simulink model "controller_template"  (Simulink 7.8)
settings: Solver=FixedStepDiscrete  SolverMode=SingleTasking  StartTime=0.0  StopTime=inf  FixedStep=Ts  RelTol=1e-3
PreLoadFcn:
  | load_waypoints
  | main;
StopFcn:
  | y_ref_wall = RecordYZ.signals(1).values(:,2);
  | y_wall = RecordYZ.signals(1).values(:,1);
  | 
  | z_ref_wall = RecordYZ.signals(2).values(:,2);
  | z_wall = RecordYZ.signals(2).values(:,1);
  | 
  | close all;
  | figure;
  | plot(y_ref_wall,z_ref_wall,'b','LineWidth',2); hold on;
  | plot(y_wall,z_wall,'r','LineWidth',2); grid on;
  | plot(traj_FG.X_ref_y_real(1,:),-traj_FG.X_ref_z_real(1,:),'o-g');
  | axis equal;
values from neighbouring files (symbols this model uses):
  Add_pitch = [0.764669359834 -6.55628329998 0 0 0.0133529191446 -0.0326334422872 0 0 0 0 0 0 ... (16 elements, 4x4)]    [kostas_malakies.mat]    (also in kostas_malakies2.mat)
  Aff_pitch = [0.764669359834 -6.55628329998 -0.0099932514458 -0.411590904828 0.0133529191446 -0.0326334422872 -8.8646944178e-05 -0.00470014240893 0 0 1 0 ... (16 elements, 4x4)]    [kostas_malakies.mat]    (also in kostas_malakies2.mat)
  Aff_roll = [0.825180563081 -6.10606264808 -0.00763580464276 -0.367448917026 0.0145694646817 0.0253169520582 -6.457583527e-05 -0.00409059128644 0 0 1 0 ... (16 elements, 4x4)]    [kostas_malakies.mat]    (also in kostas_malakies2.mat; main.m = [Aff_roll,zeros(size(Aff_roll,1),1);zeros(1,size(Aff_roll,1); main_last.m = [Aff_roll,zeros(size(Aff_roll,1),1);zeros(1,size(Aff_roll,1))
  Bdd_pitch = [0.235330640166  -0.000506747889746; 6.55628329998  -0.0141179351932; 0  0; 0  0]    [kostas_malakies.mat]    (also in kostas_malakies2.mat)
  Bff_pitch = [0.235330640166  0; 6.55628329998  0; -0.000567656018985  0; -0.0435256495914  0]    [kostas_malakies.mat]    (also in kostas_malakies2.mat)
  Bff_roll = [0.174819436919  0; 6.10606264808  0; -0.000299760068643  0; -0.0270637325616  0]    [kostas_malakies.mat]    (also in kostas_malakies2.mat; main.m = [Bff_roll;zeros(1,size(Bff_roll,2))]; main_last.m = [Bff_roll;zeros(1,size(Bff_roll,2))])
  Fi_Xdir = [-3.0499319419 0 -7.4272134917 -0.3906339295 0 0 -7.4272134917 -1.4749060606 -2.0114272215 -3.0499319419 -7.4272134917 -1.154776828 ... (624 elements, 156x4)]    [kostas_malakies.mat]    (also in kostas_malakies2.mat = [0 0 -2.6412818692 0 0 -3.3089352882 0 -2.6412818692 0 -2.64)
  Fi_XdirFF = [-0.447351940284 0 0 -1.28434394361 -4.04417159595 -1.80654990505 -1.28434394361 1 -4.04417159595 -1.80654990505 1 0 ... (536 elements, 134x4)]    [kostas_malakies.mat]    (also in kostas_malakies2.mat; matlab.mat = [-1.62441280603 -1.28434394361 -1.7723315065 -1.66810627541 )
  Fi_Yaw = [-1.14619813144 0 0]    [kostas_malakies.mat]    (also in kostas_malakies2.mat; matlab.mat = -0.284754025426)
  Fi_Ydir = [-0.466308586531 2.22044604925e-16 2.22044604925e-16 -1.46518332723 -4.54395337171 -2.00318743375 -1.46518332723 1 -4.54395337171 -2.00318743375 1 2.22044604925e-16 ... (536 elements, 134x4)]    [kostas_malakies.mat]    (also in kostas_malakies2.mat = [-0.521298425559 -2.64128186917 -15.6565978667 -8.2066553194; matlab.mat = [1 -1.9173235349 -1.46518332723 1 1 1 1 1 -1.98764774833 -1.)
  Fi_Zdir = [0 -1.80359099426e-16 0 1.4149586889 0 0 2.30859647265e-14 -5.77149118162e-15 0 0 0 0 ... (54 elements, 27x2)]    [kostas_malakies.mat]    (also in kostas_malakies2.mat = [4.30976351396 0 4.73307471514 3.80948040666 0 0 0 0.5468933; matlab.mat = [0 -9.51943523339e-14 0 1.99761158231 0 1.18992940417e-14 0 )
  g = 9.8065    [kostas_malakies.mat]    (also in kostas_malakies2.mat; load_PMModel.m = 9.81; main.m; main_last.m)
  Gi_Xdir = [33.5705355246 -0.267 268.54680224 -0.0188924328 -0.267 -0.267 268.54680224 0.039239647 0.0672163769 0.1708155012 1.343002558 0.0122735546 ... (156 elements, 156x1)]    [kostas_malakies.mat]    (also in kostas_malakies2.mat = [-0.267 -0.267 -1.8623973597 -0.267 -0.267 16.4050483477 -0.)
  Gi_XdirFF = [0 0.27 -0.27 0.478341621792 -6.42962779272 -1.98615606962 -0.478341621792 -0.373552567526 6.42962779272 1.98615606962 0.373552567526 0.27 ... (134 elements, 134x1)]    [kostas_malakies.mat]    (also in kostas_malakies2.mat; matlab.mat = [3.88578058619e-16 0.478341621792 -0.139455879222 -0.1159311)
  Gi_Yaw = [4.4408920985e-16 -3.14159265359 3.14159265359]    [kostas_malakies.mat]    (also in kostas_malakies2.mat = [-4.4408920985e-16 -3.14159265359 3.14159265359]; matlab.mat = 4.4408920985e-16)
  Gi_Ydir = [-2.77555756156e-16 0.27 -0.27 0.516209388722 7.06668201156 2.10835273651 -0.516209388722 -0.383863816771 -7.06668201156 -2.10835273651 0.383863816771 0.27 ... (134 elements, 134x1)]    [kostas_malakies.mat]    (also in kostas_malakies2.mat = [1.11022302463e-16 0.765579126644 531.260413192 11.754237275; matlab.mat = [0.383863816771 -0.133207088705 0.516209388722 0.38386381677)
  Gi_Zdir = [-1 -1 -1 2.22044604925e-16 -1 -1 -1 -1 1 -1 -1 -1 ... (27 elements, 27x1)]    [kostas_malakies.mat]    (also in kostas_malakies2.mat = [0.174387892495 -1 0.368373831608 3.33066907388e-16 -1 -1 -1; matlab.mat = [-2 -2 -2 1.11022302463e-15 -2 -2 -2 2 -2 -2 -2 2 ... (21 el)
  Hn_Xdir = [0.0894044100374 0.0185803675847 -0.0787469077295 -1 0 0.0903062437314 0.0275585020049 -0.0791302456941 -0.0894044100374 -0.0892208721324 -1 0 ... (5248 elements, 1312x4)]    [kostas_malakies.mat]    (also in kostas_malakies2.mat = [0.194772943522 -0.999280166414 0.0919386851603 -0.143548982)
  Hn_XdirFF = [-0.618529611748 0.618529611748 0.827215259158 -0.512155371354 -0.650909395739 -0.827215259158 0.930717154057 0.512155371354 0.650909395739 -0.930717154057 -1 0 ... (4464 elements, 1116x4)]    [kostas_malakies.mat]    (also in kostas_malakies2.mat; matlab.mat = [1 -0.136019433325 -0.405248495598 -0.339279056031 0 -1 0.13)
  Hn_Yaw = [1 -1 -1 1 1 -1]    [kostas_malakies.mat]    (also in kostas_malakies2.mat; matlab.mat = [1 -1])
  Hn_Ydir = [-0.642151612842 0.642151612842 0.873369621238 0.521434628645 0.668917219747 -0.873369621238 0.934789012395 -0.521434628645 -0.668917219747 -0.934789012395 -1 0 ... (4532 elements, 1133x4)]    [kostas_malakies.mat]    (also in kostas_malakies2.mat = [0.972602710123 0.0284063109089 0.559530157965 0.73050130567; matlab.mat = [0.711566553558 0.999813894311 -0.735660470031 0 0 0.5471922)
  Hn_Zdir = [-0.560552458797 -0.996815278536 -0.988320507921 0.666673243042 -1 0 -0.421994354267 -0.987440631917 -0.973284290019 -0.956170964903 -0.936236606521 0.560552458797 ... (224 elements, 112x2)]    [kostas_malakies.mat]    (also in kostas_malakies2.mat = [-0.781813705838 -0.712499731132 0.751798766698 0 -0.7286973; matlab.mat = [1 -1 -0.996815278536 -0.990718937584 -0.276007160242 0.3840)
  kalm_mpc_yaw =     [kostas_malakies.mat]    (also in kostas_malakies2.mat)
  Kn_Xdir = [0.991899150003 0.997410232697 -0.994647298545 0.5094 5 0.992251952723 0.997427328059 -0.992171068824 -0.991899150003 -0.991948411946 0.5094 5 ... (1312 elements, 1312x1)]    [kostas_malakies.mat]    (also in kostas_malakies2.mat = [0.972973501195 0.603589097273 0.988510480824 -0.97816203365)
  Kn_XdirFF = [0.373314565409 0.373314565409 0.472754204418 0.915522246067 0.951154784392 0.472754204418 0.240212330437 0.915522246067 0.951154784392 0.240212330437 0.2094 2 ... (1116 elements, 1116x1)]    [kostas_malakies.mat]    (also in kostas_malakies2.mat; matlab.mat = [0.2094 0.19132523886 0.382063154155 0.900203176458 2 0.2094)
  Kn_Yaw = [2.74088097634 2.74088097634 -2.74088097634 3.14159265359 -2.74088097634 3.14159265359]    [kostas_malakies.mat]    (also in kostas_malakies2.mat; matlab.mat = [0.0873 0.0873])
  Kn_Ydir = [0.371815875743 0.371815875743 0.451349483511 0.90366201682 0.917647772499 0.451349483511 0.24471770913 0.90366201682 0.917647772499 0.24471770913 0.2094 2 ... (1133 elements, 1133x1)]    [kostas_malakies.mat]    (also in kostas_malakies2.mat = [0.351231202126 0.997082913977 0.855763802521 0.792250278627; matlab.mat = [-0.126119149197 0.0536759032179 0.37354703421 2 2 -0.239682)
  Kn_Zdir = [0.727672356179 1.00172267683 1.00656919451 -0.471160923828 1 1 1.18526984431 1.00688561667 1.01272393898 1.01603878926 1.01572683497 -0.727672356179 ... (112 elements, 112x1)]    [kostas_malakies.mat]    (also in kostas_malakies2.mat = [0.21304012328 0.326509029469 -0.262060822346 1 0.301409884 ; matlab.mat = [1 1 1.00663007512 1.02122194908 0.632590992205 -0.384463644)
  MAX_BIAS_YAW_RATE = 0.0872664625997    [kostas_malakies.mat]    (also in kostas_malakies2.mat; main.m; main_last.m)
  Nc_Xdir = [5 10 5 15 8 13 7 11 8 9 8 8 ... (156 elements, 156x1)]    [kostas_malakies.mat]    (also in kostas_malakies2.mat = [11 10 8 9 9 7 13 7 10 7 6 12 ... (277 elements, 277x1)])
  Nc_XdirFF = [18 15 15 11 9 7 11 14 9 7 14 8 ... (134 elements, 134x1)]    [kostas_malakies.mat]    (also in kostas_malakies2.mat; matlab.mat = [14 8 7 10 8 7 10 12 10 10 12 11 ... (107 elements, 107x1)])
  Nc_Yaw = [2 2 2]    [kostas_malakies.mat]    (also in kostas_malakies2.mat; matlab.mat = 2)
  Nc_Ydir = [18 16 16 10 9 7 10 14 9 7 14 8 ... (134 elements, 134x1)]    [kostas_malakies.mat]    (also in kostas_malakies2.mat = [22 12 6 9 9 5 12 13 6 9 9 5 ... (171 elements, 171x1)]; matlab.mat = [11 8 12 15 7 9 10 13 10 14 12 7 ... (104 elements, 104x1)])
  Nc_Zdir = [6 7 3 6 3 4 4 3 6 5 3 4 ... (27 elements, 27x1)]    [kostas_malakies.mat]    (also in kostas_malakies2.mat = [4 4 3 12 5 4 3 3 4 3 3 4 ... (93 elements, 93x1)]; matlab.mat = [6 3 7 4 4 3 4 6 3 5 3 3 ... (21 elements, 21x1)])
  pitch_cmd2pitch_1stOrd = 1.42468924998    [kostas_malakies.mat]    (also in kostas_malakies2.mat)
  roll_cmd2roll_1stOrd = 1.38101661575    [kostas_malakies.mat]    (also in kostas_malakies2.mat)
  thrust_cmd2thrust_0thOrd = 0.876575459522    [kostas_malakies.mat]    (also in kostas_malakies2.mat)
  THRUST_CMD_GAIN = -0.0835    [kostas_malakies.mat]    (also in kostas_malakies2.mat; load_PMModel.m)
  traj_FG =     [kostas.mat]    (also in kostas_malakies.mat; kostas_malakies2.mat; main.m = ReferenceCreator(maxdisty,maxdistz,scale_y,scale_z); main_last.m = ReferenceCreator(maxdisty,maxdistz,scale_y,scale_z))
  Ts = 0.02    [kostas_malakies.mat]    (also in kostas_malakies2.mat; main.m; main_last.m; matlab.mat = 0.08)
  yaw_cmd2yaw_1stOrd = 2.01792090263    [kostas_malakies.mat]    (also in kostas_malakies2.mat)
  z = [-0.93079906702 -0.933865725994 -0.937557637691 -0.939011216164 -0.94143640995 -0.944628417492 -0.947235524654 -0.949601888657 -0.952827751637 -0.9567258358 -0.958320975304 -0.960991024971 ... (7988 elements, 7988x1)]    [kostas_malakies2.mat]    (also in plotDataTest.m = simout_data.signals.values(:,11))
libraries: simulink x48, Hquad_control_LIB_MPC x13
(part 2 of 3)

== system controller_template/FreeFlight Pos Ctrl/MAIN CONTROL LOOP1/demux ==
  odometry : Inport
  ref : Inport  Port=2
  reset : Inport  Port=3
  Bus Creator : BusCreator
  Bus Creator1 : BusCreator
  Bus Creator2 : BusCreator  Inputs=2
  Bus Creator3 : BusCreator  Inputs=2
  Bus Selector1 : BusSelector  OutputSignals=pose_ref.x_ref,pose_ref.y_ref,pose_ref.z_ref,pose_ref.yaw_ref
  Bus Selector2 : BusSelector  OutputSignals=rpy.pitch,ang_vel.ang_vel_y,pos.x,vel.x_dot,rpy.roll,ang_vel.ang_vel_x,pos.y,vel.y_dot,pos.z,vel.z_dot,rpy.yaw,ang_vel.ang_vel_z
  reset1 : Outport
  X_ref_x : Outport  Port=2
  x_states : Outport  Port=3
  reset2 : Outport  Port=4
  X_ref_y : Outport  Port=5
  y_states : Outport  Port=6
  reset3 : Outport  Port=7
  X_ref_z : Outport  Port=8
  z_states : Outport  Port=9
  reset4 : Outport  Port=10
  X_ref_yaw : Outport  Port=11
  yaw_states : Outport  Port=12
  wires:
  Bus Selector1/4 -> X_ref_yaw/1  "<yaw_ref>"
  Bus Selector1/3 -> X_ref_z/1  "<z_ref>"
  odometry/1 -> Bus Selector2/1
  ref/1 -> Bus Selector1/1
  Bus Selector1/1 -> X_ref_x/1  "<x_ref>"
  Bus Selector1/2 -> X_ref_y/1  "<y_ref>"
  reset/1 -> reset3/1, reset4/1, reset2/1, reset1/1
  Bus Selector2/1 -> Bus Creator/1  "<pitch>"
  Bus Selector2/2 -> Bus Creator/2  "<ang_vel_y>"
  Bus Selector2/3 -> Bus Creator/3  "<x>"
  Bus Selector2/4 -> Bus Creator/4  "<x_dot>"
  Bus Creator1/1 -> y_states/1
  Bus Selector2/5 -> Bus Creator1/1  "<roll>"
  Bus Selector2/6 -> Bus Creator1/2  "<ang_vel_x>"
  Bus Selector2/7 -> Bus Creator1/3  "<y>"
  Bus Selector2/8 -> Bus Creator1/4  "<y_dot>"
  Bus Selector2/9 -> Bus Creator2/1  "<z>"
  Bus Selector2/10 -> Bus Creator2/2  "<z_dot>"
  Bus Selector2/12 -> Bus Creator3/2  "<ang_vel_z>"
  Bus Selector2/11 -> Bus Creator3/1  "<yaw>"
  Bus Creator2/1 -> z_states/1
  Bus Creator3/1 -> yaw_states/1
  Bus Creator/1 -> x_states/1

== system controller_template/FreeFlight Pos Ctrl/MAIN CONTROL LOOP1/x controller MPC FG   ==
  reset : Inport  PortDimensions=1
  "X_ref_x  " : Inport  Port=2
  "x_states_est  " : Inport  Port=3
  Demux : Demux
  Display : Display
  Display1 : Display
  Explicit Ctrl Free Flight : Subsystem
  Explicit Ctrl Hybrid : Subsystem
  Free Flight : Subsystem
  Manual Switch : simulink/Signal Routing/Manual Switch  sw=1  action=0  varsize=off
  Manual Switch1 : simulink/Signal Routing/Manual Switch  sw=1  action=0  varsize=off
  Mean : Subsystem
  Mux : Mux
  Saturation : Saturate  UpperLimit=0.2094  LowerLimit=-0.2094
  Saturation1 : Saturate  UpperLimit=2  LowerLimit=-2
  Saturation2 : Saturate  UpperLimit=1  LowerLimit=-1
  Saturation4 : Saturate  UpperLimit=0.2094  LowerLimit=-0.2094
  Wall Deviation : Subsystem
  "pitch_cmd   " : Outport  PortDimensions=1
  x_pos : Outport  Port=2  PortDimensions=1
  wires:
  Demux/1 -> Saturation/1
  Demux/2 -> Saturation1/1
  Mux/1 -> Explicit Ctrl Hybrid/1(States), Explicit Ctrl Free Flight/1(States)
  "x_states_est  "/1 -> Demux/1
  Saturation/1 -> Mux/1
  Saturation1/1 -> Mux/2
  Saturation2/1 -> Mux/4
  Manual Switch/1 -> Mux/3, Display/1
  Mean/1(u_mean) -> "pitch_cmd   "/1, Display1/1, Explicit Ctrl Free Flight/2(input), Explicit Ctrl Hybrid/2(input)
  Saturation4/1 -> Mean/1(u)
  Demux/4 -> Saturation2/1
  Wall Deviation/1(deltax) -> Manual Switch/1
  Free Flight/1(deltax) -> Manual Switch/2
  Demux/3 -> Free Flight/1(posx), Wall Deviation/1(posx), x_pos/1
  "X_ref_x  "/1 -> Free Flight/2(refx)
  Manual Switch1/1 -> Saturation4/1
  Explicit Ctrl Hybrid/1(Input) -> Manual Switch1/1
  Explicit Ctrl Free Flight/1(Input) -> Manual Switch1/2

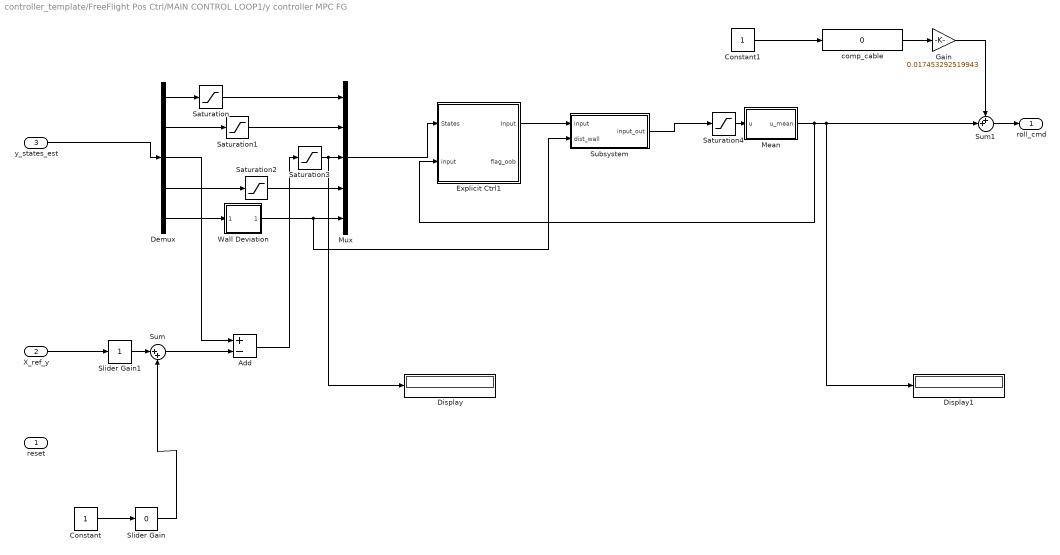
== system controller_template/FreeFlight Pos Ctrl/MAIN CONTROL LOOP1/y controller MPC FG ==
  reset : Inport  PortDimensions=1
  "X_ref_y  " : Inport  Port=2
  "y_states_est  " : Inport  Port=3
  Add : Sum  Inputs=+-
  Constant : Constant
  Constant1 : Constant
  Demux : Demux  Outputs=5
  Display : Display
  Display1 : Display
  Explicit Ctrl1 : Subsystem
  Gain : Gain  Gain=0.017453292519943
  Mean : Subsystem
  Mux : Mux  Inputs=5
  Saturation : Saturate  UpperLimit=0.2094  LowerLimit=-0.2094
  Saturation1 : Saturate  UpperLimit=2  LowerLimit=-2
  Saturation2 : Saturate  UpperLimit=1  LowerLimit=-1
  Saturation3 : Saturate  UpperLimit=1  LowerLimit=-1
  Saturation4 : Saturate  UpperLimit=0.2094  LowerLimit=-0.2094
  Slider Gain : simulink/Math Operations/Slider Gain  low=-0.4  gain=0  high=2.95
  Slider Gain1 : simulink/Math Operations/Slider Gain  low=0  gain=1  high=2.9
  Subsystem : Subsystem
  Sum : Sum  Inputs=|++
  Sum1 : Sum  Inputs=++|
  Wall Deviation : Subsystem
  comp_cable : simulink/Math Operations/Slider Gain  low=-1  gain=0  high=2
  roll_cmd : Outport  PortDimensions=1
  wires:
  Explicit Ctrl1/1(Input) -> Subsystem/1(input)
  Demux/1 -> Saturation/1
  Demux/2 -> Saturation1/1
  Demux/3 -> Add/1
  Add/1 -> Saturation3/1
  Demux/4 -> Saturation2/1
  Mux/1 -> Explicit Ctrl1/1(States)
  "y_states_est  "/1 -> Demux/1
  Saturation/1 -> Mux/1
  Saturation1/1 -> Mux/2
  Saturation2/1 -> Mux/4
  Saturation3/1 -> Mux/3, Display/1
  Mean/1(u_mean) -> Explicit Ctrl1/2(input), Display1/1, Sum1/2
  Saturation4/1 -> Mean/1(u)
  Constant/1 -> Slider Gain/1
  "X_ref_y  "/1 -> Slider Gain1/1
  Slider Gain/1 -> Sum/2
  Slider Gain1/1 -> Sum/1
  Sum/1 -> Add/2
  Demux/5 -> Wall Deviation/1(posx)
  Wall Deviation/1(deltax) -> Mux/5, Subsystem/2(dist_wall)
  Constant1/1 -> comp_cable/1
  comp_cable/1 -> Gain/1
  Gain/1 -> Sum1/1
  Sum1/1 -> roll_cmd/1
  Subsystem/1(input_out) -> Saturation4/1

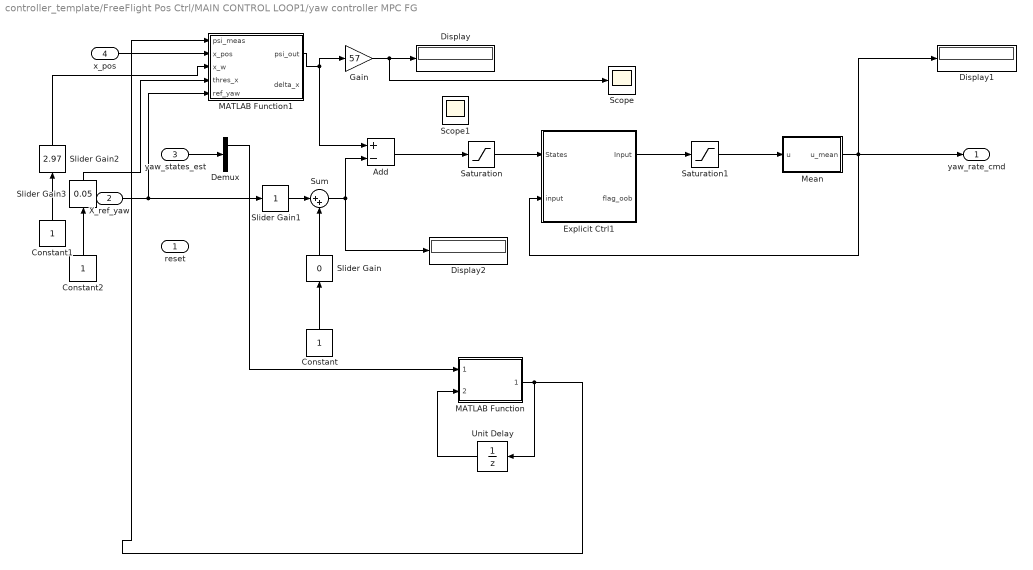
== system controller_template/FreeFlight Pos Ctrl/MAIN CONTROL LOOP1/yaw controller MPC FG ==
  reset : Inport  PortDimensions=1
  X_ref_yaw : Inport  Port=2
  "yaw_states_est  " : Inport  Port=3
  x_pos : Inport  Port=4
  Add : Sum  Inputs=+-
  Constant : Constant
  Constant1 : Constant
  Constant2 : Constant
  Demux : Demux  Outputs=2
  Display : Display
  Display1 : Display
  Display2 : Display
  Explicit Ctrl1 : Subsystem
  Gain : Gain  Gain=57
  MATLAB Function : MATLAB Function  TreatAsAtomicUnit=on
  MATLAB Function1 : MATLAB Function  TreatAsAtomicUnit=on
  Mean : Subsystem
  Saturation : Saturate  UpperLimit=pi  LowerLimit=-pi
  Saturation1 : Saturate  UpperLimit=pi  LowerLimit=-pi
  Scope : Scope
      settings: YMin=-350  YMax=50  SaveName=ScopeData21
  Scope1 : Scope
      settings: YMin=-1  YMax=5.5  SaveName=ScopeData22
  Slider Gain : simulink/Math Operations/Slider Gain  low=-0.4  gain=0  high=2.95
  Slider Gain1 : simulink/Math Operations/Slider Gain  low=0  gain=1  high=2.9
  Slider Gain2 : simulink/Math Operations/Slider Gain  low=-0.4  gain=2.97  high=2.97
  Slider Gain3 : simulink/Math Operations/Slider Gain  low=-0.4  gain=0.05  high=2.95
  Sum : Sum  Inputs=|++
  Unit Delay : UnitDelay  SampleTime=-1
  yaw_rate_cmd : Outport  PortDimensions=1
  wires:
  "yaw_states_est  "/1 -> Demux/1
  Saturation/1 -> Explicit Ctrl1/1(States)
  Explicit Ctrl1/1(Input) -> Saturation1/1
  Mean/1(u_mean) -> Explicit Ctrl1/2(input), yaw_rate_cmd/1, Display1/1
  Saturation1/1 -> Mean/1(u)
  X_ref_yaw/1 -> Slider Gain1/1, MATLAB Function1/5(ref_yaw)
  Constant/1 -> Slider Gain/1
  Slider Gain/1 -> Sum/2
  Slider Gain1/1 -> Sum/1
  Sum/1 -> Add/2, Display2/1
  Gain/1 -> Display/1, Scope/1
  MATLAB Function/1(psi_prime) -> Unit Delay/1, MATLAB Function1/1(psi_meas)
  Unit Delay/1 -> MATLAB Function/2(psi_prev)
  Demux/1 -> MATLAB Function/1(psi_meas)
  Add/1 -> Saturation/1
  x_pos/1 -> MATLAB Function1/2(x_pos)
  MATLAB Function1/1(psi_out) -> Gain/1, Add/1
  Constant1/1 -> Slider Gain2/1
  Slider Gain2/1 -> MATLAB Function1/3(x_w)
  Constant2/1 -> Slider Gain3/1
  Slider Gain3/1 -> MATLAB Function1/4(thres_x)

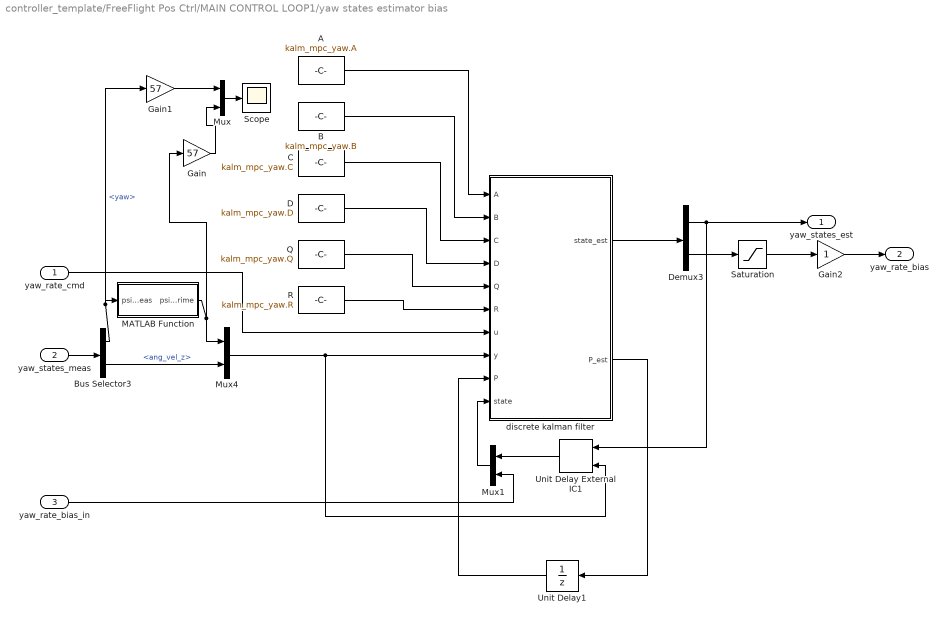
== system controller_template/FreeFlight Pos Ctrl/MAIN CONTROL LOOP1/yaw states estimator bias ==
  yaw_rate_cmd : Inport  PortDimensions=1
  yaw_states_meas : Inport  Port=2  PortDimensions=2
  yaw_rate_bias_in : Inport  Port=3  PortDimensions=1
  A : Constant  Value=kalm_mpc_yaw.A
  B : Constant  Value=kalm_mpc_yaw.B
  Bus Selector3 : BusSelector  OutputSignals=yaw,ang_vel_z
  C : Constant  Value=kalm_mpc_yaw.C
  D : Constant  Value=kalm_mpc_yaw.D
  Demux3 : Demux  Outputs=2
  Gain : Gain  Gain=57
  Gain1 : Gain  Gain=57
  Gain2 : Gain
  MATLAB Function : MATLAB Function  TreatAsAtomicUnit=on
  Mux : Mux  Inputs=2
  Mux1 : Mux  Inputs=2
  Mux4 : Mux  Inputs=2
  Q : Constant  Value=kalm_mpc_yaw.Q
  R : Constant  Value=kalm_mpc_yaw.R
  Saturation : Saturate  UpperLimit=MAX_BIAS_YAW_RATE  LowerLimit=-MAX_BIAS_YAW_RATE
  Scope : Scope
      settings: YMin=-225  YMax=200  SaveName=ScopeData23
  Unit Delay External IC1 : simulink/Additional Math & Discrete/Additional Discrete/Unit Delay External IC  tsamp=-1
  Unit Delay1 : UnitDelay  X0=kalm_mpc_yaw.P  SampleTime=Ts
  discrete kalman filter : MATLAB Function  AncestorBlock=Hquad_control_LIB_LQRI/x states estimator/discrete kalman filter  TreatAsAtomicUnit=on
  yaw_states_est : Outport  PortDimensions=2
  yaw_rate_bias : Outport  Port=2  PortDimensions=1
  wires:
  Unit Delay External IC1/1 -> Mux1/1
  yaw_rate_bias_in/1 -> Mux1/2
  Mux1/1 -> discrete kalman filter/10(state)
  Saturation/1 -> Gain2/1
  Demux3/1 -> Unit Delay External IC1/1, yaw_states_est/1
  Demux3/2 -> Saturation/1
  R/1 -> discrete kalman filter/6(R)
  Q/1 -> discrete kalman filter/5(Q)
  Mux4/1 -> discrete kalman filter/8(y), Unit Delay External IC1/2
  yaw_rate_cmd/1 -> discrete kalman filter/7(u)
  Unit Delay1/1 -> discrete kalman filter/9(P)
  discrete kalman filter/2(P_est) -> Unit Delay1/1
  discrete kalman filter/1(state_est) -> Demux3/1
  D/1 -> discrete kalman filter/4(D)
  C/1 -> discrete kalman filter/3(C)
  B/1 -> discrete kalman filter/2(B)
  A/1 -> discrete kalman filter/1(A)
  yaw_states_meas/1 -> Bus Selector3/1
  Bus Selector3/1 -> MATLAB Function/1(psi_meas), Gain1/1  "<yaw>"
  Bus Selector3/2 -> Mux4/2  "<ang_vel_z>"
  MATLAB Function/1(psi_prime) -> Mux4/1, Gain/1
  Mux/1 -> Scope/1
  Gain/1 -> Mux/2
  Gain1/1 -> Mux/1
  Gain2/1 -> yaw_rate_bias/1

== system controller_template/FreeFlight Pos Ctrl/MAIN CONTROL LOOP1/z controller MPC FG ==
  reset : Inport  PortDimensions=1
  X_ref_z : Inport  Port=2
  "z_states_est  " : Inport  Port=3
  Add : Sum  Inputs=+-
  Demux : Demux  Outputs=3
  Display : Display
  Display1 : Display
  Explicit Ctrl1 : Subsystem
  Mean : Subsystem
  Mux : Mux  Inputs=3
  Saturation : Saturate  UpperLimit=1  LowerLimit=-1
  Saturation1 : Saturate  UpperLimit=1  LowerLimit=-1
  Saturation2 : Saturate  UpperLimit=1  LowerLimit=-1
  Slider Gain : simulink/Math Operations/Slider Gain  low=0  gain=1.1  high=2
  Subsystem : Subsystem
  Wall Deviation : Subsystem
  thrust_cmd : Outport  PortDimensions=1
  wires:
  "z_states_est  "/1 -> Demux/1
  Demux/2 -> Saturation/1
  Demux/1 -> Add/1
  X_ref_z/1 -> Add/2
  Add/1 -> Saturation1/1
  Mux/1 -> Explicit Ctrl1/1(States)
  Saturation/1 -> Mux/2
  Saturation1/1 -> Display/1, Mux/1, Subsystem/3(dz)
  Mean/1(u_mean) -> thrust_cmd/1, Display1/1
  Saturation2/1 -> Mean/1(u)
  Demux/3 -> Wall Deviation/1(posx)
  Wall Deviation/1(deltax) -> Mux/3, Subsystem/2(dx)
  Explicit Ctrl1/1(Input) -> Subsystem/1(u_thrust)
  Subsystem/1(u_thrust_out) -> Slider Gain/1
  Slider Gain/1 -> Saturation2/1

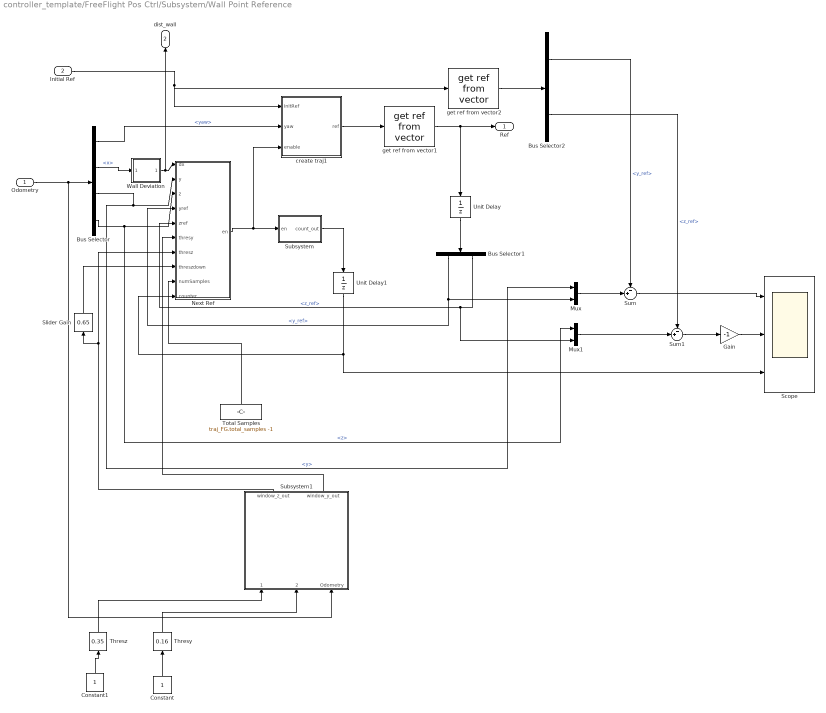
== system controller_template/FreeFlight Pos Ctrl/Subsystem/Wall Point Reference ==
  Odometry : Inport
  Initial Ref : Inport  Port=2
  Bus Selector : BusSelector  OutputSignals=rpy.yaw,pos.x,pos.y,pos.z
  Bus Selector1 : BusSelector  OutputSignals=pose_ref.y_ref,pose_ref.z_ref
  Bus Selector2 : BusSelector  OutputSignals=pose_ref.y_ref,pose_ref.z_ref
  Constant : Constant
  Constant1 : Constant
  Gain : Gain  Gain=-1
  Mux : Mux  Inputs=2
  Mux1 : Mux  Inputs=2
  Next Ref : MATLAB Function  TreatAsAtomicUnit=on
  Scope : Scope  NumInputPorts=3
      settings: YMin=-0.05~0.45~58  YMax=0.4~0.63~64  SaveName=RecordYZ
  Slider Gain : simulink/Math Operations/Slider Gain  low=0  gain=0.65  high=2
  Subsystem : Subsystem
  Subsystem1 : Subsystem
  Sum : Sum  Inputs=-+|
  Sum1 : Sum  Inputs=-+|
  Thresy : simulink/Math Operations/Slider Gain  low=0  gain=0.16  high=1
  Thresz : simulink/Math Operations/Slider Gain  low=0  gain=0.35  high=2
  Total Samples : Constant  Value=traj_FG.total_samples -1
  Unit Delay : UnitDelay  SampleTime=-1
  Unit Delay1 : UnitDelay  SampleTime=-1
  Wall Deviation : Subsystem
  create traj1 : Subsystem
  get ref from vector1 : Hquad_control_LIB_MPC/pos controller/get ref from vector
  get ref from vector2 : Hquad_control_LIB_MPC/pos controller/get ref from vector
  Ref : Outport
  dist_wall : Outport  Port=2
  wires:
  get ref from vector1/1 -> Ref/1, Unit Delay/1
  create traj1/1(ref) -> get ref from vector1/1
  Initial Ref/1 -> create traj1/1(InitRef), get ref from vector2/1
  Odometry/1 -> Bus Selector/1, Subsystem1/3(Odometry)
  Bus Selector/1 -> create traj1/2(yaw)  "<yaw>"
  Bus Selector/3 -> Next Ref/2(y), Mux/1  "<y>"
  Bus Selector/4 -> Next Ref/3(z), Mux1/1  "<z>"
  Unit Delay/1 -> Bus Selector1/1
  Bus Selector1/1 -> Next Ref/4(yref), Mux/2  "<y_ref>"
  Bus Selector1/2 -> Next Ref/5(zref), Mux1/2  "<z_ref>"
  Constant/1 -> Thresy/1
  Thresy/1 -> Subsystem1/2(nominal_window_y)
  Next Ref/1(en) -> create traj1/3(enable), Subsystem/1(en)
  Wall Deviation/1(deltax) -> Next Ref/1(dx), dist_wall/1
  Bus Selector/2 -> Wall Deviation/1(posx)  "<x>"
  Total Samples/1 -> Next Ref/9(numSamples)
  Unit Delay1/1 -> Next Ref/10(counter), Scope/3
  Subsystem/1(count_out) -> Unit Delay1/1
  Constant1/1 -> Thresz/1
  Thresz/1 -> Subsystem1/1(nominal_window_z)
  Gain/1 -> Scope/2
  Mux/1 -> Sum/2
  Mux1/1 -> Sum1/2
  Sum1/1 -> Gain/1
  Sum/1 -> Scope/1
  get ref from vector2/1 -> Bus Selector2/1
  Bus Selector2/1 -> Sum/1  "<y_ref>"
  Bus Selector2/2 -> Sum1/1  "<z_ref>"
  Subsystem1/2(window_y_out) -> Next Ref/6(thresy)
  Subsystem1/1(window_z_out) -> Next Ref/7(thresz), Slider Gain/1
  Slider Gain/1 -> Next Ref/8(threszdown)

== system controller_template/FreeFlight Pos Ctrl/decoupling and rotation/decoupling  ==
  "roll_meas  " : Inport  PortDimensions=1
  "pitch_meas  " : Inport  Port=2  PortDimensions=1
  cmd : Inport  Port=3
  mass : Inport  Port=4
  posx : Inport  Port=5
  Bus Creator : BusCreator
  Bus Selector3 : BusSelector  OutputSignals=pitch_cmd,roll_cmd,thrust_cmd,yaw_rate_cmd
  Embedded MATLAB Function : MATLAB Function  TreatAsAtomicUnit=on
  Wall Deviation : Subsystem
  g : Constant  Value=g
  "cmd_comp  " : Outport
  wires:
  "roll_meas  "/1 -> Embedded MATLAB Function/2(roll_meas)
  "pitch_meas  "/1 -> Embedded MATLAB Function/1(pitch_meas)
  cmd/1 -> Bus Selector3/1
  Bus Selector3/4 -> Bus Creator/4  "<yaw_rate_cmd>"
  Bus Creator/1 -> "cmd_comp  "/1
  Embedded MATLAB Function/3(thrust_comp) -> Bus Creator/3  "thrust_cmd"
  Embedded MATLAB Function/2(roll_cmd_comp) -> Bus Creator/2  "roll_cmd"
  Embedded MATLAB Function/1(pitch_cmd_comp) -> Bus Creator/1  "pitch_cmd"
  Bus Selector3/1 -> Embedded MATLAB Function/3(pitch_cmd)  "<pitch_cmd>"
  Bus Selector3/2 -> Embedded MATLAB Function/4(roll_cmd)  "<roll_cmd>"
  Bus Selector3/3 -> Embedded MATLAB Function/5(thrust)  "<thrust_cmd>"
  mass/1 -> Embedded MATLAB Function/6(m)
  g/1 -> Embedded MATLAB Function/7(g)
  posx/1 -> Wall Deviation/1(posx)
  Wall Deviation/1(deltax) -> Embedded MATLAB Function/8(posx)

== system controller_template/FreeFlight Pos Ctrl/decoupling and rotation/rotate_to_quat_frame ==
  yaw_meas : Inport
  cmd_comp : Inport  Port=2
  bias : Inport  Port=3
  Bus Creator1 : BusCreator
  Bus Creator2 : BusCreator
  Bus Selector1 : BusSelector  OutputSignals=thrust_bias,yaw_rate_bias
  Bus Selector2 : BusSelector  OutputSignals=pitch_bias,roll_bias
  Bus Selector3 : BusSelector  OutputSignals=pitch_cmd,roll_cmd
  Bus Selector4 : BusSelector  OutputSignals=thrust_cmd,yaw_rate_cmd
  Embedded MATLAB Function : MATLAB Function  TreatAsAtomicUnit=on
  "cmd_rot  " : Outport
  bias_rot : Outport  Port=2
  wires:
  yaw_meas/1 -> Embedded MATLAB Function/1(yaw)
  bias/1 -> Bus Selector2/1, Bus Selector1/1
  Bus Creator1/1 -> bias_rot/1
  Bus Selector2/1 -> Embedded MATLAB Function/4(pitch_bias)  "<pitch_bias>"
  Bus Selector2/2 -> Embedded MATLAB Function/5(roll_bias)  "<roll_bias>"
  Embedded MATLAB Function/3(pitch_bias_rot) -> Bus Creator1/1  "pitch_bias"
  Embedded MATLAB Function/4(roll_bias_rot) -> Bus Creator1/2  "roll_bias"
  Bus Creator2/1 -> "cmd_rot  "/1
  Bus Selector3/2 -> Embedded MATLAB Function/3(roll_cmd)  "<roll_cmd>"
  Bus Selector3/1 -> Embedded MATLAB Function/2(pitch_cmd)  "<pitch_cmd>"
  cmd_comp/1 -> Bus Selector3/1, Bus Selector4/1
  Embedded MATLAB Function/1(pitch_rot) -> Bus Creator2/1  "pitch_cmd"
  Embedded MATLAB Function/2(roll_rot) -> Bus Creator2/2  "roll_cmd"
  Bus Selector4/1 -> Bus Creator2/3  "<thrust_cmd>"
  Bus Selector4/2 -> Bus Creator2/4  "<yaw_rate_cmd>"
  Bus Selector1/1 -> Bus Creator1/3  "<thrust_bias>"
  Bus Selector1/2 -> Bus Creator1/4  "<yaw_rate_bias>"

== system controller_template/pos controller/MAIN CONTROL LOOP1/demux ==
  odometry : Inport
  ref : Inport  Port=2
  reset : Inport  Port=3
  Bus Creator : BusCreator  Inputs=3
  Bus Creator1 : BusCreator  Inputs=3
  Bus Creator2 : BusCreator  Inputs=2
  Bus Creator3 : BusCreator  Inputs=2
  Bus Selector1 : BusSelector  OutputSignals=X_ref_x,X_ref_y,X_ref_z,X_ref_yaw
  Bus Selector2 : BusSelector  OutputSignals=pos.x,vel.x_dot,rpy.pitch,pos.y,vel.y_dot,rpy.roll,pos.z,vel.z_dot,rpy.yaw,ang_vel.ang_vel_z
  reset1 : Outport
  X_ref_x : Outport  Port=2
  x_states_meas : Outport  Port=3  PortDimensions=3
  reset2 : Outport  Port=4
  X_ref_y : Outport  Port=5
  y_states_meas : Outport  Port=6  PortDimensions=3
  reset3 : Outport  Port=7
  X_ref_z : Outport  Port=8
  z_states_meas : Outport  Port=9  PortDimensions=2
  reset4 : Outport  Port=10
  X_ref_yaw : Outport  Port=11
  yaw_states_meas : Outport  Port=12  PortDimensions=2
  wires:
  Bus Selector1/4 -> X_ref_yaw/1  "<X_ref_yaw>"
  Bus Selector1/3 -> X_ref_z/1  "<X_ref_z>"
  Bus Selector2/6 -> Bus Creator1/3  "<roll>"
  Bus Selector2/3 -> Bus Creator/3  "<pitch>"
  odometry/1 -> Bus Selector2/1
  Bus Creator/1 -> x_states_meas/1
  Bus Selector2/1 -> Bus Creator/1  "<x>"
  Bus Selector2/2 -> Bus Creator/2  "<x_dot>"
  Bus Selector2/4 -> Bus Creator1/1  "<y>"
  Bus Selector2/5 -> Bus Creator1/2  "<y_dot>"
  Bus Creator1/1 -> y_states_meas/1
  Bus Selector2/7 -> Bus Creator2/1  "<z>"
  Bus Selector2/8 -> Bus Creator2/2  "<z_dot>"
  Bus Selector2/9 -> Bus Creator3/1  "<yaw>"
  Bus Selector2/10 -> Bus Creator3/2  "<ang_vel_z>"
  Bus Creator2/1 -> z_states_meas/1
  Bus Creator3/1 -> yaw_states_meas/1
  ref/1 -> Bus Selector1/1
  Bus Selector1/1 -> X_ref_x/1  "<X_ref_x>"
  Bus Selector1/2 -> X_ref_y/1  "<X_ref_y>"
  reset/1 -> reset3/1, reset4/1, reset2/1, reset1/1

== system controller_template/pos controller/MAIN CONTROL LOOP1/yaw states estimator bias ==
  yaw_rate_cmd : Inport  PortDimensions=1
  yaw_states_meas : Inport  Port=2  PortDimensions=2
  yaw_rate_bias_in : Inport  Port=3  PortDimensions=1
  A : Constant  Value=kalm_mpc_yaw.A
  B : Constant  Value=kalm_mpc_yaw.B
  Bus Selector3 : BusSelector  OutputSignals=yaw,ang_vel_z
  C : Constant  Value=kalm_mpc_yaw.C
  D : Constant  Value=kalm_mpc_yaw.D
  Demux3 : Demux  Outputs=2
  Mux1 : Mux  Inputs=2
  Mux4 : Mux  Inputs=2
  Q : Constant  Value=kalm_mpc_yaw.Q
  R : Constant  Value=kalm_mpc_yaw.R
  Saturation : Saturate  UpperLimit=MAX_BIAS_YAW_RATE  LowerLimit=-MAX_BIAS_YAW_RATE
  Unit Delay External IC1 : simulink/Additional Math & Discrete/Additional Discrete/Unit Delay External IC  tsamp=-1
  Unit Delay1 : UnitDelay  X0=kalm_mpc_yaw.P  SampleTime=Ts
  discrete kalman filter : MATLAB Function  AncestorBlock=Hquad_control_LIB_LQRI/x states estimator/discrete kalman filter  TreatAsAtomicUnit=on
  yaw_states_est : Outport  PortDimensions=2
  yaw_rate_bias : Outport  Port=2  PortDimensions=1
  wires:
  Unit Delay External IC1/1 -> Mux1/1
  yaw_rate_bias_in/1 -> Mux1/2
  Mux1/1 -> discrete kalman filter/10(state)
  Saturation/1 -> yaw_rate_bias/1
  Demux3/1 -> yaw_states_est/1, Unit Delay External IC1/1
  Demux3/2 -> Saturation/1
  R/1 -> discrete kalman filter/6(R)
  Q/1 -> discrete kalman filter/5(Q)
  Mux4/1 -> discrete kalman filter/8(y), Unit Delay External IC1/2
  yaw_rate_cmd/1 -> discrete kalman filter/7(u)
  Unit Delay1/1 -> discrete kalman filter/9(P)
  discrete kalman filter/2(P_est) -> Unit Delay1/1
  discrete kalman filter/1(state_est) -> Demux3/1
  D/1 -> discrete kalman filter/4(D)
  C/1 -> discrete kalman filter/3(C)
  B/1 -> discrete kalman filter/2(B)
  A/1 -> discrete kalman filter/1(A)
  yaw_states_meas/1 -> Bus Selector3/1
  Bus Selector3/1 -> Mux4/1  "<yaw>"
  Bus Selector3/2 -> Mux4/2  "<ang_vel_z>"

== system controller_template/FreeFlight Pos Ctrl/MAIN CONTROL LOOP1/x controller MPC FG  /Explicit Ctrl Free Flight ==
  States : Inport
  input : Inport  Port=2
  Constant5 : Constant  Value=Hn_XdirFF
  Constant6 : Constant  Value=Kn_XdirFF
  Constant7 : Constant  Value=Fi_XdirFF
  Constant8 : Constant  Value=Gi_XdirFF
  Constant9 : Constant  Value=Nc_XdirFF
  Ctrl_Xdir : MATLAB Function  TreatAsAtomicUnit=on
  PitchPropagateFF : Subsystem
  Rate Transition : RateTransition  OutPortSampleTime=0.08
  Rate Transition1 : RateTransition  OutPortSampleTime=0.08
  Unit Delay2 : UnitDelay  SampleTime=-1
  Input : Outport
  flag_oob : Outport  Port=2
  wires:
  Ctrl_Xdir/2(flag_oob) -> flag_oob/1
  Ctrl_Xdir/1(U) -> Input/1
  States/1 -> Rate Transition/1
  Unit Delay2/1 -> PitchPropagateFF/1(uprev)
  Rate Transition/1 -> PitchPropagateFF/2(x)
  input/1 -> Rate Transition1/1
  Rate Transition1/1 -> Unit Delay2/1
  PitchPropagateFF/1(Out1) -> Ctrl_Xdir/1(X)
  Constant9/1 -> Ctrl_Xdir/6(Nc)
  Constant8/1 -> Ctrl_Xdir/5(Gi)
  Constant7/1 -> Ctrl_Xdir/4(Fi)
  Constant6/1 -> Ctrl_Xdir/3(Kn)
  Constant5/1 -> Ctrl_Xdir/2(Hn)

== system controller_template/FreeFlight Pos Ctrl/MAIN CONTROL LOOP1/x controller MPC FG  /Explicit Ctrl Hybrid ==
  States : Inport
  input : Inport  Port=2
  Constant : Constant  Value=Hn_Xdir
  Constant1 : Constant  Value=Kn_Xdir
  Constant2 : Constant  Value=Fi_Xdir
  Constant4 : Constant  Value=Nc_Xdir
  Constat3 : Constant  Value=Gi_Xdir
  Ctrl_Xdir : MATLAB Function  TreatAsAtomicUnit=on
  PitchPropagate : Subsystem
  Rate Transition : RateTransition  OutPortSampleTime=0.08
  Rate Transition1 : RateTransition  OutPortSampleTime=0.08
  Unit Delay2 : UnitDelay  SampleTime=-1
  Input : Outport
  flag_oob : Outport  Port=2
  wires:
  Ctrl_Xdir/2(flag_oob) -> flag_oob/1
  Ctrl_Xdir/1(U) -> Input/1
  States/1 -> Rate Transition/1
  Unit Delay2/1 -> PitchPropagate/1(uprev)
  Rate Transition/1 -> PitchPropagate/2(x)
  input/1 -> Rate Transition1/1
  Rate Transition1/1 -> Unit Delay2/1
  PitchPropagate/1(Out1) -> Ctrl_Xdir/1(X)
  Constant/1 -> Ctrl_Xdir/2(Hn)
  Constant1/1 -> Ctrl_Xdir/3(Kn)
  Constant2/1 -> Ctrl_Xdir/4(Fi)
  Constat3/1 -> Ctrl_Xdir/5(Gi)
  Constant4/1 -> Ctrl_Xdir/6(Nc)

== system controller_template/FreeFlight Pos Ctrl/MAIN CONTROL LOOP1/x controller MPC FG  /Free Flight ==
  posx : Inport
  refx : Inport  Port=2
  Add : Sum  Inputs=+-
  Saturation3 : Saturate  UpperLimit=1  LowerLimit=-1
  deltax : Outport
  wires:
  posx/1 -> Add/1
  Add/1 -> Saturation3/1
  Saturation3/1 -> deltax/1
  refx/1 -> Add/2

== system controller_template/FreeFlight Pos Ctrl/MAIN CONTROL LOOP1/x controller MPC FG  /Mean ==
  u : Inport
  Gain : Gain  Gain=.33333
  Sum : Sum  Inputs=|++
  Sum1 : Sum  Inputs=|++
  Unit Delay : UnitDelay  SampleTime=-1
  Unit Delay1 : UnitDelay  SampleTime=-1
  Unit Delay2 : UnitDelay  SampleTime=-1
  u_mean : Outport
  wires:
  u/1 -> Sum/1
  Sum/1 -> Gain/1
  Gain/1 -> u_mean/1, Unit Delay1/1, Unit Delay2/1
  Unit Delay1/1 -> Unit Delay/1
  Unit Delay/1 -> Sum1/2
  Sum1/1 -> Sum/2
  Unit Delay2/1 -> Sum1/1

== system controller_template/FreeFlight Pos Ctrl/MAIN CONTROL LOOP1/x controller MPC FG  /Wall Deviation ==
  posx : Inport
  Add : Sum  Inputs=+-
  Constant : Constant
  Constant1 : Constant
  MATLAB Function : MATLAB Function  TreatAsAtomicUnit=on
  Saturation3 : Saturate  UpperLimit=0  LowerLimit=-1
  Slider Gain : simulink/Math Operations/Slider Gain  low=-0.4  gain=2.589  high=3
  Slider Gain1 : simulink/Math Operations/Slider Gain  low=-0.4  gain=2.97  high=3
  Slider Gain2 : simulink/Math Operations/Slider Gain  low=-0.4  gain=-0.05  high=2.95
  deltax : Outport
  wires:
  posx/1 -> Add/1
  Constant1/1 -> Slider Gain2/1
  Slider Gain2/1 -> MATLAB Function/2(thres)
  Add/1 -> MATLAB Function/1(u)
  MATLAB Function/1(y) -> Saturation3/1
  Saturation3/1 -> deltax/1
  Constant/1 -> Slider Gain/1
  Slider Gain/1 -> Add/2

== system controller_template/FreeFlight Pos Ctrl/MAIN CONTROL LOOP1/y controller MPC FG/Explicit Ctrl1 ==
  States : Inport
  input : Inport  Port=2
  Constant : Constant  Value=Hn_Ydir
  Constant1 : Constant  Value=Kn_Ydir
  Constant2 : Constant  Value=Fi_Ydir
  Constant3 : Constant  Value=Gi_Ydir
  Constant4 : Constant  Value=Nc_Ydir
  Ctrl_Xdir : MATLAB Function  TreatAsAtomicUnit=on
  Rate Transition : RateTransition  OutPortSampleTime=0.08
  Rate Transition1 : RateTransition  OutPortSampleTime=0.08
  RollPropagate : Subsystem
  Unit Delay2 : UnitDelay  SampleTime=-1
  Input : Outport
  flag_oob : Outport  Port=2
  wires:
  Ctrl_Xdir/2(flag_oob) -> flag_oob/1
  Ctrl_Xdir/1(U) -> Input/1
  Constant4/1 -> Ctrl_Xdir/6(Nc)
  Constant3/1 -> Ctrl_Xdir/5(Gi)
  Constant2/1 -> Ctrl_Xdir/4(Fi)
  Constant1/1 -> Ctrl_Xdir/3(Kn)
  Constant/1 -> Ctrl_Xdir/2(Hn)
  States/1 -> Rate Transition/1
  input/1 -> Rate Transition1/1
  Rate Transition1/1 -> Unit Delay2/1
  Unit Delay2/1 -> RollPropagate/1(uprev)
  RollPropagate/1(Out1) -> Ctrl_Xdir/1(X)
  Rate Transition/1 -> RollPropagate/2(x)

== system controller_template/FreeFlight Pos Ctrl/MAIN CONTROL LOOP1/y controller MPC FG/Mean ==
  u : Inport
  Gain : Gain  Gain=.33333
  Sum : Sum  Inputs=|++
  Sum1 : Sum  Inputs=|++
  Unit Delay : UnitDelay  SampleTime=-1
  Unit Delay1 : UnitDelay  SampleTime=-1
  Unit Delay2 : UnitDelay  SampleTime=-1
  u_mean : Outport
  wires:
  u/1 -> Sum/1
  Sum/1 -> Gain/1
  Gain/1 -> u_mean/1, Unit Delay1/1, Unit Delay2/1
  Unit Delay1/1 -> Unit Delay/1
  Unit Delay/1 -> Sum1/2
  Sum1/1 -> Sum/2
  Unit Delay2/1 -> Sum1/1

== system controller_template/FreeFlight Pos Ctrl/MAIN CONTROL LOOP1/y controller MPC FG/Subsystem ==
  input : Inport
  dist_wall : Inport  Port=2
  Constant : Constant
  MATLAB Function : MATLAB Function  TreatAsAtomicUnit=on
  Slider Gain2 : simulink/Math Operations/Slider Gain  low=0  gain=1.5  high=2
  input_out : Outport
  wires:
  input/1 -> MATLAB Function/1(input)
  dist_wall/1 -> MATLAB Function/2(dist_wall)
  Slider Gain2/1 -> MATLAB Function/3(K_gain)
  Constant/1 -> Slider Gain2/1
  MATLAB Function/1(input_out) -> input_out/1

== system controller_template/FreeFlight Pos Ctrl/MAIN CONTROL LOOP1/y controller MPC FG/Wall Deviation ==
  posx : Inport
  Add : Sum  Inputs=+-
  Constant : Constant
  Constant1 : Constant
  MATLAB Function : MATLAB Function  TreatAsAtomicUnit=on
  Saturation3 : Saturate  UpperLimit=0.1  LowerLimit=-1
  Slider Gain : simulink/Math Operations/Slider Gain  low=-0.4  gain=2.97  high=3
  Slider Gain2 : simulink/Math Operations/Slider Gain  low=-0.4  gain=-0.07  high=2.95
  deltax : Outport
  wires:
  posx/1 -> Add/1
  Constant1/1 -> Slider Gain2/1
  Slider Gain2/1 -> MATLAB Function/2(thres)
  Add/1 -> MATLAB Function/1(u)
  MATLAB Function/1(y) -> Saturation3/1
  Saturation3/1 -> deltax/1
  Constant/1 -> Slider Gain/1
  Slider Gain/1 -> Add/2

== system controller_template/FreeFlight Pos Ctrl/MAIN CONTROL LOOP1/yaw controller MPC FG/Explicit Ctrl1 ==
  States : Inport
  input : Inport  Port=2
  Constant : Constant  Value=Hn_Yaw
  Constant1 : Constant  Value=Kn_Yaw
  Constant2 : Constant  Value=Fi_Yaw
  Constant3 : Constant  Value=Gi_Yaw
  Constant4 : Constant  Value=Nc_Yaw
  Ctrl_Xdir : MATLAB Function  TreatAsAtomicUnit=on
  Display : Display
  Rate Transition : RateTransition  OutPortSampleTime=0.02
  Rate Transition1 : RateTransition  OutPortSampleTime=0.02
  Unit Delay2 : UnitDelay  SampleTime=-1
  YawPropagate : Subsystem
  Input : Outport
  flag_oob : Outport  Port=2
  wires:
  Ctrl_Xdir/2(flag_oob) -> flag_oob/1
  Ctrl_Xdir/1(U) -> Input/1
  Constant4/1 -> Ctrl_Xdir/6(Nc)
  Constant3/1 -> Ctrl_Xdir/5(Gi)
  Constant2/1 -> Ctrl_Xdir/4(Fi)
  Constant1/1 -> Ctrl_Xdir/3(Kn)
  Constant/1 -> Ctrl_Xdir/2(Hn)
  States/1 -> Rate Transition/1
  Unit Delay2/1 -> YawPropagate/1(uprev)
  Rate Transition/1 -> YawPropagate/2(x)
  YawPropagate/1(Out1) -> Ctrl_Xdir/1(X), Display/1
  input/1 -> Rate Transition1/1
  Rate Transition1/1 -> Unit Delay2/1

== system controller_template/FreeFlight Pos Ctrl/MAIN CONTROL LOOP1/yaw controller MPC FG/Mean ==
  u : Inport
  Gain : Gain  Gain=.33333
  Sum : Sum  Inputs=|++
  Sum1 : Sum  Inputs=|++
  Unit Delay : UnitDelay  SampleTime=-1
  Unit Delay1 : UnitDelay  SampleTime=-1
  Unit Delay2 : UnitDelay  SampleTime=-1
  u_mean : Outport
  wires:
  u/1 -> Sum/1
  Sum/1 -> Gain/1
  Gain/1 -> u_mean/1, Unit Delay1/1, Unit Delay2/1
  Unit Delay1/1 -> Unit Delay/1
  Unit Delay/1 -> Sum1/2
  Sum1/1 -> Sum/2
  Unit Delay2/1 -> Sum1/1

== system controller_template/FreeFlight Pos Ctrl/MAIN CONTROL LOOP1/z controller MPC FG/Explicit Ctrl1 ==
  States : Inport
  Constant : Constant  Value=Hn_Zdir
  Constant1 : Constant  Value=Kn_Zdir
  Constant2 : Constant  Value=Fi_Zdir
  Constant3 : Constant  Value=Gi_Zdir
  Constant4 : Constant  Value=Nc_Zdir
  Ctrl_Xdir : MATLAB Function  TreatAsAtomicUnit=on
  Rate Transition : RateTransition  OutPortSampleTime=Tsz
  Input : Outport
  flag_oob : Outport  Port=2
  wires:
  Ctrl_Xdir/2(flag_oob) -> flag_oob/1
  Rate Transition/1 -> Ctrl_Xdir/1(X)
  Ctrl_Xdir/1(U) -> Input/1
  Constant4/1 -> Ctrl_Xdir/6(Nc)
  Constant3/1 -> Ctrl_Xdir/5(Gi)
  Constant2/1 -> Ctrl_Xdir/4(Fi)
  Constant1/1 -> Ctrl_Xdir/3(Kn)
  Constant/1 -> Ctrl_Xdir/2(Hn)
  States/1 -> Rate Transition/1

== system controller_template/FreeFlight Pos Ctrl/MAIN CONTROL LOOP1/z controller MPC FG/Mean ==
  u : Inport
  Gain : Gain  Gain=.33333
  Sum : Sum  Inputs=|++
  Sum1 : Sum  Inputs=|++
  Unit Delay : UnitDelay  SampleTime=-1
  Unit Delay1 : UnitDelay  SampleTime=-1
  Unit Delay2 : UnitDelay  SampleTime=-1
  u_mean : Outport
  wires:
  u/1 -> Sum/1
  Sum/1 -> Gain/1
  Gain/1 -> u_mean/1, Unit Delay1/1, Unit Delay2/1
  Unit Delay1/1 -> Unit Delay/1
  Unit Delay/1 -> Sum1/2
  Sum1/1 -> Sum/2
  Unit Delay2/1 -> Sum1/1

== system controller_template/FreeFlight Pos Ctrl/MAIN CONTROL LOOP1/z controller MPC FG/Subsystem ==
  u_thrust : Inport
  dx : Inport  Port=2
  dz : Inport  Port=3
  Constant : Constant
  MATLAB Function : MATLAB Function  TreatAsAtomicUnit=on
  Slider Gain : simulink/Math Operations/Slider Gain  low=0  gain=1  high=2
  u_thrust_out : Outport
  wires:
  u_thrust/1 -> MATLAB Function/1(u_thrust)
  dx/1 -> MATLAB Function/2(dx)
  dz/1 -> MATLAB Function/3(dz)
  Slider Gain/1 -> MATLAB Function/4(K_g_up)
  Constant/1 -> Slider Gain/1
  MATLAB Function/1(u_thrust_out) -> u_thrust_out/1

== system controller_template/FreeFlight Pos Ctrl/MAIN CONTROL LOOP1/z controller MPC FG/Wall Deviation ==
  posx : Inport
  Add : Sum  Inputs=+-
  Constant : Constant
  Constant1 : Constant
  MATLAB Function : MATLAB Function  TreatAsAtomicUnit=on
  Saturation3 : Saturate  UpperLimit=.1  LowerLimit=-1
  Slider Gain : simulink/Math Operations/Slider Gain  low=-0.4  gain=2.97  high=3
  Slider Gain2 : simulink/Math Operations/Slider Gain  low=-0.4  gain=-0.07  high=2.95
  deltax : Outport
  wires:
  posx/1 -> Add/1
  Constant1/1 -> Slider Gain2/1
  Slider Gain2/1 -> MATLAB Function/2(thres)
  Add/1 -> MATLAB Function/1(u)
  MATLAB Function/1(y) -> Saturation3/1
  Saturation3/1 -> deltax/1
  Constant/1 -> Slider Gain/1
  Slider Gain/1 -> Add/2

== system controller_template/FreeFlight Pos Ctrl/Subsystem/Wall Point Reference/Subsystem ==
  en : Inport
  MATLAB Function : MATLAB Function  TreatAsAtomicUnit=on
  Unit Delay : UnitDelay  SampleTime=-1
  Unit Delay1 : UnitDelay  SampleTime=-1
  count_out : Outport
  wires:
  en/1 -> MATLAB Function/1(en_flag), Unit Delay/1
  Unit Delay/1 -> MATLAB Function/2(en_flag_prev)
  MATLAB Function/1(count_out) -> Unit Delay1/1, count_out/1
  Unit Delay1/1 -> MATLAB Function/3(count_out_prev)

== system controller_template/FreeFlight Pos Ctrl/Subsystem/Wall Point Reference/Subsystem1 ==
  nominal_window_z : Inport
  nominal_window_y : Inport  Port=2
  Odometry : Inport  Port=3
  Bus Selector : BusSelector  OutputSignals=vel.z_dot,vel.y_dot
  Constant{,1..3} (4 alike) : Constant
  MATLAB Function : MATLAB Function  TreatAsAtomicUnit=on
  Scope : Scope  NumInputPorts=2
      settings: YMin=0.3~0.15  YMax=0.3~0.15  SaveName=ScopeData16
  Slider Gain : simulink/Math Operations/Slider Gain  low=0  gain=0.0515  high=2
  Slider Gain1 : simulink/Math Operations/Slider Gain  low=0  gain=10.065  high=10.065
  Slider Gain2 : simulink/Math Operations/Slider Gain  low=0  gain=1  high=2
  Slider Gain3 : simulink/Math Operations/Slider Gain  low=0  gain=0.095  high=2
  Slider Gain4 : simulink/Math Operations/Slider Gain  low=0  gain=0  high=2
  Switch : Switch  Threshold=0.5
  Switch1 : Switch  Threshold=0.5
  window_z_out : Outport
  window_y_out : Outport  Port=2
  wires:
  nominal_window_z/1 -> MATLAB Function/1(nominal_window_z), Switch/3
  nominal_window_y/1 -> MATLAB Function/2(nominal_window_y), Switch1/3
  Slider Gain/1 -> MATLAB Function/5(thres_vel_z)
  Constant/1 -> Slider Gain/1, Slider Gain1/1
  Slider Gain1/1 -> MATLAB Function/6(thres_vel_y)
  Slider Gain2/1 -> MATLAB Function/7(K_gain)
  Constant1/1 -> Slider Gain2/1
  Slider Gain3/1 -> MATLAB Function/8(maxDeltaWindow)
  Constant2/1 -> Slider Gain3/1
  MATLAB Function/1(nominal_window_z_out) -> Switch/1
  Switch/1 -> window_z_out/1, Scope/1
  MATLAB Function/2(nominal_window_y_out) -> Switch1/1
  Switch1/1 -> window_y_out/1, Scope/2
  Constant3/1 -> Slider Gain4/1
  Slider Gain4/1 -> Switch/2, Switch1/2
  Odometry/1 -> Bus Selector/1
  Bus Selector/1 -> MATLAB Function/3(vel_z)  "<z_dot>"
  Bus Selector/2 -> MATLAB Function/4(vel_y)  "<y_dot>"

== system controller_template/FreeFlight Pos Ctrl/Subsystem/Wall Point Reference/Wall Deviation ==
  posx : Inport
  Add : Sum  Inputs=+-
  Constant : Constant
  Constant1 : Constant
  MATLAB Function : MATLAB Function  TreatAsAtomicUnit=on
  Saturation3 : Saturate  UpperLimit=0  LowerLimit=-1
  Slider Gain : simulink/Math Operations/Slider Gain  low=-0.4  gain=2.97  high=3
  Slider Gain2 : simulink/Math Operations/Slider Gain  low=-0.4  gain=-0.07  high=2.95
  deltax : Outport
  wires:
  posx/1 -> Add/1
  Constant1/1 -> Slider Gain2/1
  Slider Gain2/1 -> MATLAB Function/2(thres)
  Add/1 -> MATLAB Function/1(u)
  MATLAB Function/1(y) -> Saturation3/1
  Saturation3/1 -> deltax/1
  Constant/1 -> Slider Gain/1
  Slider Gain/1 -> Add/2

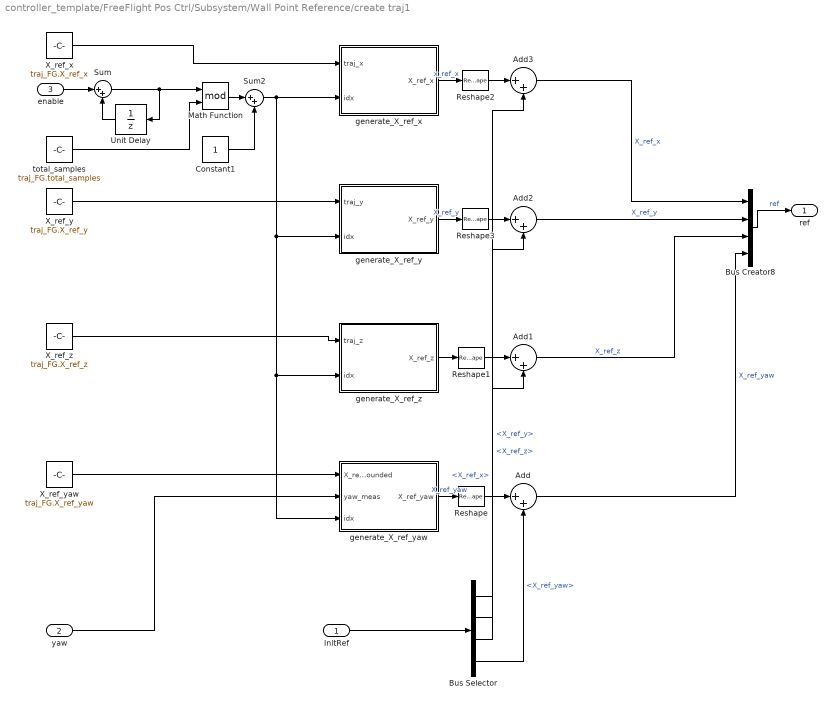
== system controller_template/FreeFlight Pos Ctrl/Subsystem/Wall Point Reference/create traj1 ==
  InitRef : Inport
  yaw : Inport  Port=2
  enable : Inport  Port=3
  Add{,1..3} (4 alike) : Sum  Inputs=|++
  Bus Creator8 : BusCreator
  Bus Selector : BusSelector  OutputSignals=X_ref_x,X_ref_y,X_ref_z,X_ref_yaw
  Constant1 : Constant
  Math Function : Math  Operator=mod  SaturateOnIntegerOverflow=on
  Reshape{,1..3} (4 alike) : Reshape
  Sum : Sum  Inputs=|++
  Sum2 : Sum  Inputs=|++
  Unit Delay : UnitDelay  SampleTime=-1
  X_ref_x : Constant  Value=traj_FG.X_ref_x
  X_ref_y : Constant  Value=traj_FG.X_ref_y
  X_ref_yaw : Constant  Value=traj_FG.X_ref_yaw
  X_ref_z : Constant  Value=traj_FG.X_ref_z
  generate_X_ref_x : MATLAB Function  TreatAsAtomicUnit=on
  generate_X_ref_y : MATLAB Function  TreatAsAtomicUnit=on
  generate_X_ref_yaw : MATLAB Function  TreatAsAtomicUnit=on
  generate_X_ref_z : MATLAB Function  TreatAsAtomicUnit=on
  total_samples : Constant  Value=traj_FG.total_samples
  ref : Outport
  wires:
  Bus Creator8/1 -> ref/1  "ref"
  enable/1 -> Sum/1
  Unit Delay/1 -> Sum/2
  Sum/1 -> Unit Delay/1, Math Function/1
  total_samples/1 -> Math Function/2
  Math Function/1 -> Sum2/1
  Constant1/1 -> Sum2/2
  yaw/1 -> generate_X_ref_yaw/2(yaw_meas)
  Sum2/1 -> generate_X_ref_x/2(idx), generate_X_ref_yaw/3(idx), generate_X_ref_z/2(idx), generate_X_ref_y/2(idx)
  X_ref_y/1 -> generate_X_ref_y/1(traj_y)
  X_ref_x/1 -> generate_X_ref_x/1(traj_x)
  X_ref_yaw/1 -> generate_X_ref_yaw/1(X_ref_yaw_unbounded)
  X_ref_z/1 -> generate_X_ref_z/1(traj_z)
  InitRef/1 -> Bus Selector/1
  generate_X_ref_yaw/1(X_ref_yaw) -> Reshape/1  "X_ref_yaw"
  Add/1 -> Bus Creator8/4  "X_ref_yaw"
  generate_X_ref_x/1(X_ref_x) -> Reshape2/1  "x_ref_x"
  Add3/1 -> Bus Creator8/1  "X_ref_x"
  generate_X_ref_y/1(X_ref_y) -> Reshape3/1  "X_ref_y"
  Add2/1 -> Bus Creator8/2  "X_ref_y"
  generate_X_ref_z/1(X_ref_z) -> Reshape1/1
  Add1/1 -> Bus Creator8/3  "X_ref_z"
  Bus Selector/4 -> Add/2  "<X_ref_yaw>"
  Bus Selector/3 -> Add1/2  "<X_ref_z>"
  Bus Selector/2 -> Add2/2  "<X_ref_y>"
  Bus Selector/1 -> Add3/2  "<X_ref_x>"
  Reshape2/1 -> Add3/1
  Reshape3/1 -> Add2/1
  Reshape1/1 -> Add1/1
  Reshape/1 -> Add/1

== system controller_template/FreeFlight Pos Ctrl/decoupling and rotation/decoupling /Wall Deviation ==
  posx : Inport
  Add : Sum  Inputs=+-
  Constant : Constant
  Constant1 : Constant
  MATLAB Function : MATLAB Function  TreatAsAtomicUnit=on
  Saturation3 : Saturate  UpperLimit=0  LowerLimit=-1
  Slider Gain : simulink/Math Operations/Slider Gain  low=-0.4  gain=2.97  high=3
  Slider Gain2 : simulink/Math Operations/Slider Gain  low=-0.4  gain=-0.05  high=2.95
  deltax : Outport
  wires:
  posx/1 -> Add/1
  Constant1/1 -> Slider Gain2/1
  Slider Gain2/1 -> MATLAB Function/2(thres)
  Add/1 -> MATLAB Function/1(u)
  MATLAB Function/1(y) -> Saturation3/1
  Saturation3/1 -> deltax/1
  Constant/1 -> Slider Gain/1
  Slider Gain/1 -> Add/2

== system controller_template/FreeFlight Pos Ctrl/MAIN CONTROL LOOP1/x controller MPC FG  /Explicit Ctrl Free Flight/PitchPropagateFF ==
  uprev : Inport
  x : Inport  Port=2
  Constant : Constant  Value=Aff_pitch
  Constant1 : Constant  Value=Bff_pitch
  Demux : Demux
  MATLAB Function : MATLAB Function  TreatAsAtomicUnit=on
  Mux : Mux
  Saturation : Saturate  UpperLimit=0.2094  LowerLimit=-0.2094
  Saturation1 : Saturate  UpperLimit=2  LowerLimit=-2
  Saturation2 : Saturate  UpperLimit=1  LowerLimit=-1
  Saturation3 : Saturate  UpperLimit=1  LowerLimit=-1
  Out1 : Outport
  wires:
  uprev/1 -> MATLAB Function/4(u)
  Mux/1 -> Out1/1
  Saturation/1 -> Mux/1
  Saturation1/1 -> Mux/2
  Saturation2/1 -> Mux/4
  Saturation3/1 -> Mux/3
  MATLAB Function/1(y) -> Demux/1
  Demux/1 -> Saturation/1
  Demux/2 -> Saturation1/1
  Demux/3 -> Saturation3/1
  Demux/4 -> Saturation2/1
  Constant1/1 -> MATLAB Function/3(B)
  Constant/1 -> MATLAB Function/2(A)
  x/1 -> MATLAB Function/1(x)
